simulink model "model"  (R2019a)
settings: Solver=VariableStepAuto  StartTime=0.0  StopTime=10.0  RelTol=1e-3
undefined symbols (not defined in the file): m
libraries: simulink x4
settings Model: Creator=jacoboffersen  LastModifiedBy=jacoboffersen

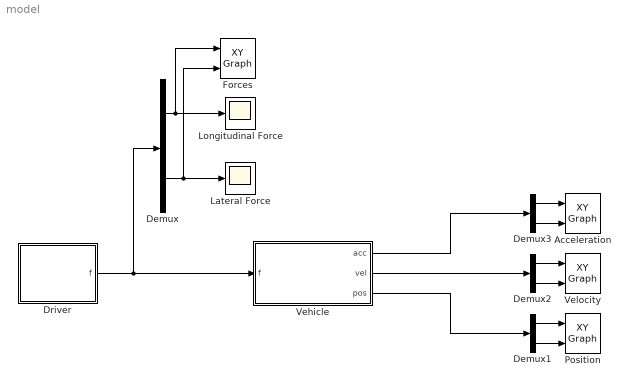
== system model ==
  Acceleration : simulink/Sinks/XY Graph  xmin=-1  xmax=1  ymin=-1  ymax=1  st=-1
  Demux{,1..3} (4 alike) : Demux  Outputs=2
  Driver : Subsystem
  Forces : simulink/Sinks/XY Graph  xmin=-1  xmax=1  ymin=-1  ymax=1  st=-1
  Lateral Force : Scope
  Longitudinal Force : Scope
  Position : simulink/Sinks/XY Graph  xmin=-1  xmax=1  ymin=-1  ymax=1  st=-1
  Vehicle : Subsystem
  Velocity : simulink/Sinks/XY Graph  xmin=-1  xmax=1  ymin=-1  ymax=1  st=-1
  wires:
  Driver/1(f) -> Demux/1, Vehicle/1(f)
  Demux/2 -> Forces/2, Lateral Force/1
  Demux/1 -> Forces/1, Longitudinal Force/1
  Demux1/2 -> Position/2
  Demux1/1 -> Position/1
  Demux2/1 -> Velocity/1
  Demux3/1 -> Acceleration/1
  Demux3/2 -> Acceleration/2
  Demux2/2 -> Velocity/2
  Vehicle/1(acc) -> Demux3/1
  Vehicle/2(vel) -> Demux2/1
  Vehicle/3(pos) -> Demux1/1

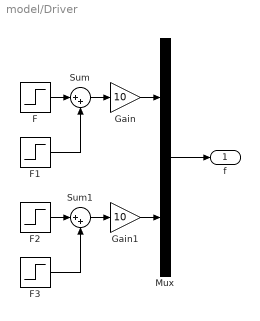
== system model/Driver ==
  F : Step  Time=2  SampleTime=0
  F1 : Step  Time=4  After=-1  SampleTime=0
  F2 : Step  Time=6  SampleTime=0
  F3 : Step  Time=8  After=-1  SampleTime=0
  Gain : Gain  Gain=10
  Gain1 : Gain  Gain=10
  Mux : Mux  Inputs=2
  Sum : Sum  Inputs=|++
  Sum1 : Sum  Inputs=|++
  f : Outport
  wires:
  F1/1 -> Sum/2
  F/1 -> Sum/1
  F3/1 -> Sum1/2
  F2/1 -> Sum1/1
  Sum/1 -> Gain/1
  Sum1/1 -> Gain1/1
  Mux/1 -> f/1
  Gain/1 -> Mux/1
  Gain1/1 -> Mux/2

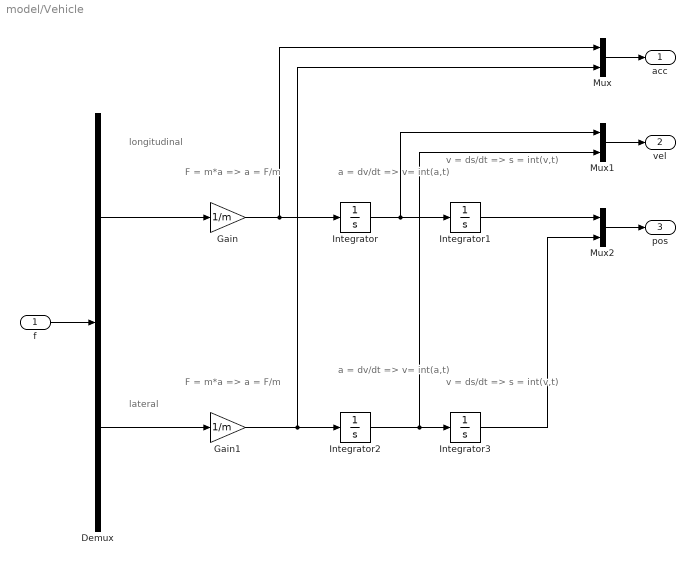
== system model/Vehicle ==
  note: lateral
  note: longitudinal
  note: a = dv/dt =>
      | v= int(a,t)
  note: v = ds/dt =>
      | s = int(v,t)
  note: F = m*a =>
      | a = F/m
  note: v = ds/dt =>
      | s = int(v,t)
  note: a = dv/dt =>
      | v= int(a,t)
  note: F = m*a =>
      | a = F/m
  f : Inport
  Demux : Demux  Outputs=2
  Gain : Gain  Gain=1/m
  Gain1 : Gain  Gain=1/m
  Integrator{,1..3} (4 alike) : Integrator
  Mux : Mux  Inputs=2
  Mux1 : Mux  Inputs=2
  Mux2 : Mux  Inputs=2
  acc : Outport
  vel : Outport  Port=2
  pos : Outport  Port=3
  wires:
  Integrator/1 -> Mux1/1, Integrator1/1
  Gain/1 -> Mux/1, Integrator/1
  f/1 -> Demux/1
  Demux/1 -> Gain/1
  Gain1/1 -> Mux/2, Integrator2/1
  Demux/2 -> Gain1/1
  Integrator2/1 -> Mux1/2, Integrator3/1
  Mux/1 -> acc/1
  Mux1/1 -> vel/1
  Mux2/1 -> pos/1
  Integrator1/1 -> Mux2/1
  Integrator3/1 -> Mux2/2
